simulink model "integratoin_2"  (R2023b)
settings: Solver=FixedStepAuto  StartTime=0.0  StopTime=inf  FixedStep=Ts  RelTol=1e-3
InitFcn:
  | params
  | pin_params
undefined symbols (not defined in the file): b, den_Gd, encoder_scale, f, J, Kb, KD, Kf, KI, Km, KP, l, L, num_Gd, r, R, Vlim, Wref
libraries: arduinolib x29, arduinosensorlib x12, simulink x8
(part 1 of 2)
settings Model: SimulationMode=external  ExtModeTrigDuration=2  Creator=SJ  LastModifiedBy=SJ
settings SolverCC: AutoInsertRateTranBlk=on
settings OptimizationCC: EnhancedBackFolding=on  PassReuseOutputArgsAs=Individual arguments  ZeroExternalMemoryAtStartup=off  ZeroInternalMemoryAtStartup=off  MaxStackSize=64  OptimizeBlockOrder=speed  DifferentSizesBufferReuse=on  OptimizationCustomize=off  EfficientTunableParamExpr=on
settings DebuggingCC: MultiTaskRateTransMsg=warning  ParameterTunabilityLossMsg=error
settings HardwareCC: ProdBitPerInt=16  ProdBitPerPointer=16  ProdBitPerSizeT=16  ProdBitPerPtrDiffT=16  ProdLargestAtomicFloat=None  ProdWordSize=8  ProdHWDeviceType=Atmel->AVR
settings SFSimCC: MATLABDynamicMemAlloc=off
settings RTWCC: Description=Embedded Coder  SystemTargetFile=ert.tlc  HardwareBoard=Arduino Mega 2560  TemplateMakefile=ert_default_tmf  Toolchain=Arduino AVR  BuildConfiguration=Faster Runs
settings CodeAppCC: ForceParamTrailComments=on  IgnoreCustomStorageClasses=off  OperatorAnnotations=on  SimulinkDataObjDesc=on  SFDataObjDesc=on  InsertBlockDesc=on
settings ERTTargetCC: SupportContinuousTime=on  SupportVariableSizeSignals=on  ExtMode=on  ExtModeTransport=3  ExtModeStaticAlloc=on  ExtModeAutomaticAllocSize=off  ExtModeStaticAllocSize=2048  ExtModeMexFile=ext_xcp  ExtModeMexArgs=0 3 921600  ExtModeIntrfLevel=Level2 - Open

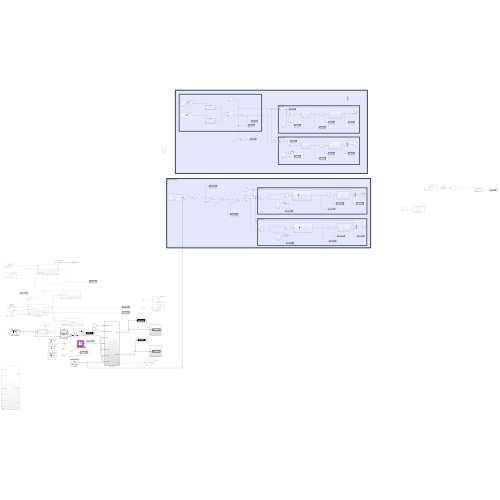
[thumbnail: Simulink's stored preview of the top-level diagram]
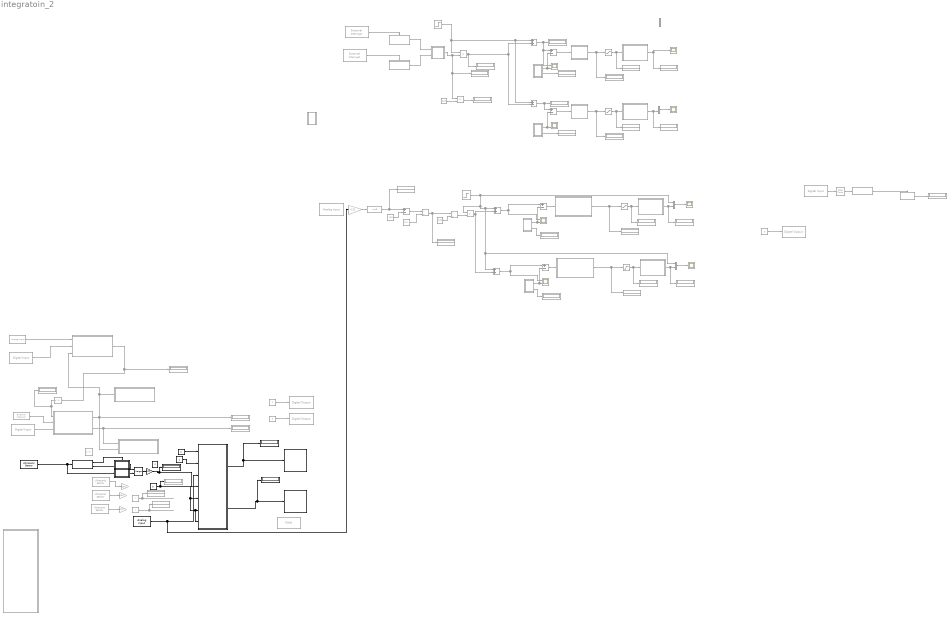
== system integratoin_2 ==
  note: Left Motor
  note: Left Motor
  note: Right Motor
  note: Variable resistance
  note: sw1,2로 1퍼 증가, 감소
  note: Right Motor
  note: 조도 센서 값 * 0.25
      | (평상시 값 800 초반, 손으로 가렸을 때 값 200~300)
  Add : Sum  Commented=on
  Add{1..3,5,7..8} (6 alike) : Sum  Commented=on  Inputs=+-
  Add4 : Sum  Commented=on
  Add6 : Sum  Commented=on
  Analog Input : arduinolib/Analog Input  Commented=on  pinNumber=8  ReadResultsOnly=off  ConversionTriggerSource=Software  ExternalTriggerType=uint32( 0 )  OutputDataType=uint16  EnableConversionCompleteNotify=off  EnableOuputStatus=off  SampleTime=-1  blockPlatform=arduino
  Analog Input1 : arduinolib/Analog Input  Commented=on  pinNumber=BS  ReadResultsOnly=off  ConversionTriggerSource=Software  ExternalTriggerType=uint32( 0 )  OutputDataType=uint16  EnableConversionCompleteNotify=off  EnableOuputStatus=off  SampleTime=-1  blockPlatform=arduino
  Chart : Stateflow chart  Commented=on  TreatAsAtomicUnit=on
  Constant : Constant  Commented=on  Value=128
  Constant1 : Constant  Commented=on  Value=6.4
  Constant10 : Constant  Commented=on  Value=0
  Constant11 : Constant
  Constant12 : Constant
  Constant2 : Constant  Commented=on  Value=100
  Constant3 : Constant  Commented=on  Value=100
  Constant4 : Constant  Value=f
  Constant5 : Constant  Commented=on  Value=0
  Constant6 : Constant  Commented=on  Value=r
  Constant7 : Constant  Value=b
  Constant8 : Constant  Commented=on  Value=l
  Constant9 : Constant  Commented=on
  Data Type Conversion : DataTypeConversion  Commented=on  OutDataTypeStr=uint8  SaturateOnIntegerOverflow=off  RndMeth=Floor
  Delay : Delay  Commented=on  DelayLength=1
  Delay1 : Delay  Commented=on  DelayLength=1
  Digital Input : arduinolib/Digital Input  Commented=on  pinNumber=20  mode=Default  Direction=input  SampleTime=0.1  blockPlatform=arduino
  Digital Input1 : arduinolib/Digital Input  Commented=on  pinNumber=SW3  mode=Default  Direction=input  SampleTime=0.1  blockPlatform=arduino
  Digital Input2 : arduinolib/Digital Input  Commented=on  pinNumber=SW2  mode=Default  Direction=input  SampleTime=0.1  blockPlatform=arduino
  Display{,1..25,29..31,33..34} (31 alike) : Display  Commented=on
  Display27 : Display
  Display28 : Display
  Display32 : Display
  Divide : Product  Commented=on  Inputs=**
  Divide1 : Product  Commented=on  Inputs=*/
  Divide2 : Product  Commented=on  Inputs=**
  Divide3 : Product  Commented=on  Inputs=*/
  Divide4 : Product  Commented=on  Inputs=**
  External Interrupt : arduinolib/External Interrupt  Commented=on  Pin=20  PullUp=off  Mode=FALLING  InterruptSimulationInput=off
  External Interrupt1 : arduinolib/External Interrupt  Commented=on  Pin=21  PullUp=off  Mode=FALLING  InterruptSimulationInput=off
  External Interrupt2 : arduinolib/External Interrupt  Commented=on  Pin=2  PullUp=off  Mode=RISING  InterruptSimulationInput=off
  Function-Call Subsystem1 : Subsystem  Commented=on  TreatAsAtomicUnit=on
  Function-Call Subsystem4 : Subsystem  Commented=on  TreatAsAtomicUnit=on
  Gain : Gain  Commented=on  Gain=0.25
  Gain1 : Gain  Gain=100
  Gain2 : Gain  Commented=on  Gain=100
  Gain3 : Gain  Commented=on  Gain=100
  Gain4 : Gain  Commented=on  Gain=100
  If : If  Commented=on  IfExpression=u1 == 0  ShowElse=off
  If Action Subsystem : Subsystem  Commented=on  TreatAsAtomicUnit=on
  If Action Subsystem1 : Subsystem  TreatAsAtomicUnit=on
  If Action Subsystem2 : Subsystem  TreatAsAtomicUnit=on
  If1 : If  IfExpression=u1 > 1
  LED_B Ctrl : Subsystem  Commented=on
  LED_R Ctrl : Subsystem  Commented=on
  L_Motor(시계) : arduinolib/Digital Output  Commented=on  pinNumber=Motor_L_Direction  Direction=output  blockPlatform=arduino
  Merge : Merge
  Mux{1..4} (4 alike) : Mux  Commented=on  Inputs=2
  PWM1 : arduinolib/PWM  Commented=on  pinNumber=Buzzer  frequencyType=Default  desiredFrequency=490.2  achievableFrequency=490.2
  R_Motor(반시계) : arduinolib/Digital Output  Commented=on  pinNumber=Motor_R_Direction  Direction=output  blockPlatform=arduino
  R_Motor(반시계)1 : arduinolib/Digital Output  Commented=on  pinNumber=Motor_R_Direction  Direction=output  blockPlatform=arduino
  Rate Transition : RateTransition  Commented=on  OutPortSampleTime=0.5
  Saturation{,1..3} (4 alike) : Saturate  Commented=on  UpperLimit=12  LowerLimit=0
  Scope{,1,4,6} (4 alike) : Scope  Commented=on  NumInputPorts=2
  Scope{2..3,5,7} (4 alike) : Scope  Commented=on
  State_Ctrl : Subsystem  Commented=on
  Step : Step  Commented=on  After=Wref  SampleTime=0
  Step1 : Step  Commented=on  After=Wref  SampleTime=0
  Subsystem : Subsystem  Commented=on
  Subsystem1 : Subsystem  Commented=on
  Subsystem10 : Subsystem  Commented=on
  Subsystem11 : Subsystem  Commented=on
  Subsystem12 : Subsystem  Commented=on
  Subsystem13 : Subsystem  Commented=on
  Subsystem14 : Subsystem
  Subsystem15 : Subsystem
  Subsystem16 : Subsystem
  Subsystem2 : Subsystem  Commented=on
  Subsystem3 : Subsystem  Commented=on
  Subsystem4 : Subsystem  Commented=on
  Subsystem5 : Subsystem  Commented=on
  Subsystem6 : Subsystem  Commented=on
  Subsystem7 : Subsystem  Commented=on
  Subsystem8 : Subsystem  Commented=on
  Subsystem9 : Subsystem  Commented=on
  light_Ctrl : Subsystem  Commented=on
  가변저항 : arduinolib/Analog Input  pinNumber=VR  ReadResultsOnly=off  ConversionTriggerSource=Software  ExternalTriggerType=uint32( 0 )  OutputDataType=uint16  EnableConversionCompleteNotify=off  EnableOuputStatus=off  SampleTime=-1  blockPlatform=arduino
  우측 초음파 : arduinosensorlib/Ultrasonic Sensor  Commented=on  NumSignalPins=2  TrigPin=R_Triger  EchoPin=R_Echo  SignalPin=3  SampleTime_=0.1  blockPlatform=ARDUINO
  전방 초음파 : arduinosensorlib/Ultrasonic Sensor  NumSignalPins=2  TrigPin=F_Triger  EchoPin=F_Echo  SignalPin=3  SampleTime_=0.01  blockPlatform=ARDUINO
  좌측 초음파 : arduinosensorlib/Ultrasonic Sensor  Commented=on  NumSignalPins=2  TrigPin=L_Triger  EchoPin=L_Echo  SignalPin=3  SampleTime_=0.1  blockPlatform=ARDUINO
  후방 초음파 : arduinosensorlib/Ultrasonic Sensor  Commented=on  NumSignalPins=2  TrigPin=B_Triger  EchoPin=B_Echo  SignalPin=3  SampleTime_=0.1  blockPlatform=ARDUINO
  wires:
  Subsystem/1(Out1) -> Add1/2, Scope/2
  Saturation/1 -> Subsystem1/1(In2), Display/1
  Subsystem1/1(Out1) -> Scope3/1, Display3/1
  External Interrupt/1 -> Function-Call Subsystem4/Trigger
  External Interrupt1/1 -> Function-Call Subsystem1/Trigger
  Function-Call Subsystem4/1(sw1) -> Chart/1(sw1)
  Function-Call Subsystem1/1(sw2) -> Chart/2(sw2)
  Step/1 -> Divide/1, Add8/1, Add/1
  Divide/1 -> Display1/1, Add/2, Add8/2
  Chart/1(n) -> Divide4/1, Display7/1, Divide/2
  Subsystem/2(Out2) -> Display5/1
  Gain/1 -> Data Type Conversion/1
  Step1/1 -> Mux2/1, Add6/1, Mux3/1, Add4/1, Divide2/1
  Data Type Conversion/1 -> Display12/1, Add2/1
  Constant/1 -> Add2/2
  Divide1/1 -> Display6/1, Divide3/1
  Add2/1 -> Divide1/1
  Constant1/1 -> Divide1/2
  Divide2/1 -> Add6/2, Add4/2
  Constant2/1 -> Divide3/2
  Divide3/1 -> Divide2/2
  Add/1 -> Scope/1, Add1/1, Display4/1
  Saturation1/1 -> Subsystem4/1(In2), Display8/1
  Subsystem3/2(Out2) -> Display11/1
  Subsystem3/1(Out1) -> Add3/2, Scope1/2
  Subsystem4/1(Out1) -> Display10/1, Mux2/2
  Mux2/1 -> Scope2/1
  Add4/1 -> Add3/1, Scope1/1
  Subsystem5/1(Out1) -> Display9/1, Saturation1/1
  Add3/1 -> Subsystem5/1(In1)
  Subsystem6/1(Out1) -> Display2/1, Saturation/1
  Add1/1 -> Subsystem6/1(In1)
  Add6/1 -> Add5/1, Scope4/1
  Mux3/1 -> Scope5/1
  Subsystem7/2(Out2) -> Display14/1
  Subsystem8/1(Out1) -> Display13/1, Mux3/2
  Subsystem7/1(Out1) -> Add5/2, Scope4/2
  Add5/1 -> Subsystem9/1(In1)
  Saturation2/1 -> Subsystem8/1(In2), Display15/1
  Subsystem9/1(Out1) -> Display16/1, Saturation2/1
  Add7/1 -> Subsystem12/1(In1)
  Subsystem11/1(Out1) -> Display19/1, Mux4/2
  Saturation3/1 -> Subsystem11/1(In2), Display17/1
  Mux4/1 -> Scope7/1
  Subsystem10/1(Out1) -> Add7/2, Scope6/2
  Subsystem12/1(Out1) -> Display18/1, Saturation3/1
  Subsystem10/2(Out2) -> Display20/1
  Add8/1 -> Add7/1, Display21/1
  Divide4/1 -> Display22/1
  Constant3/1 -> Divide4/2
  Digital Input/1 -> Rate Transition/1
  If/1 -> If Action Subsystem/Action
  If Action Subsystem/1(Out1) -> Display23/1
  Rate Transition/1 -> If/1
  Constant5/1 -> R_Motor(반시계)/1
  Constant10/1 -> R_Motor(반시계)1/1
  후방 초음파/1 -> Gain2/1
  좌측 초음파/1 -> Gain3/1
  State_Ctrl/1(Drive_mode) -> Display24/1, light_Ctrl/3(Drive_mode1), LED_R Ctrl/1(Drive_mode), LED_B Ctrl/2(Drive_mode)
  Digital Input2/1 -> State_Ctrl/3(SW2)
  Constant9/1 -> L_Motor(시계)/1
  Constant6/1 -> Display29/1
  Analog Input1/1 -> light_Ctrl/1(light1)
  Delay/1 -> Display34/1, State_Ctrl/1(light_mode)
  ? -> PWM1/1
  Digital Input1/1 -> light_Ctrl/2(In2)
  우측 초음파/1 -> Gain4/1
  Constant7/1 -> Subsystem14/7(우측 초음파), Subsystem14/6(좌측 초음파), Subsystem14/5(전방 초음파), Display31/1
  State_Ctrl/2(ADAS_state1) -> LED_B Ctrl/1(ADAS_state), Display25/1
  Constant8/1 -> Display30/1
  가변저항/1 -> Subsystem14/3(가변저항), Gain/1
  External Interrupt2/1 -> State_Ctrl/2(SW1)
  light_Ctrl/1(light_mode) -> Display33/1, Delay/1
  Constant11/1 -> Subsystem14/1(DRIVE MODE)
  Constant12/1 -> Subsystem14/2(ADAS MODE)
  If1/1 -> If Action Subsystem1/Action
  If Action Subsystem1/1(Out1) -> Merge/1
  Merge/1 -> Gain1/1
  If1/2 -> If Action Subsystem2/Action
  If Action Subsystem2/1(Out1) -> Merge/2
  Subsystem14/1(L_Motor) -> Subsystem15/1(L_Motor), Display27/1
  Subsystem14/2(R_Motor) -> Display28/1, Subsystem16/1(L_Motor)
  Gain1/1 -> Subsystem14/4(In1), Display32/1
  ? -> ?
  ? -> ?
  전방 초음파/1 -> If Action Subsystem2/1(In1), If1/1

== system integratoin_2/Function-Call Subsystem1 ==
  function : TriggerPort  TriggerType=function-call  VariantControl=(inherit)
  Add : Sum  Inputs=+-
  Constant : Constant
  Delay : Delay  DelayLength=1
  sw2 : Outport
  wires:
  Add/1 -> Delay/1, sw2/1
  Delay/1 -> Add/2
  Constant/1 -> Add/1

== system integratoin_2/Function-Call Subsystem4 ==
  function : TriggerPort  TriggerType=function-call  VariantControl=(inherit)
  Add : Sum  Inputs=+-
  Constant : Constant
  Delay : Delay  DelayLength=1
  sw1 : Outport
  wires:
  Add/1 -> sw1/1, Delay/1
  Delay/1 -> Add/2
  Constant/1 -> Add/1

== system integratoin_2/If Action Subsystem ==
  Action Port : ActionPort  ActionPortLabel=if(u1 == 0)
  Add : Sum
  Constant : Constant
  Constant1 : Constant  Value=3
  Delay : Delay  DelayLength=1
  Mod : Math  Operator=mod
  Out1 : Outport
  wires:
  Mod/1 -> Delay/1, Out1/1
  Delay/1 -> Add/2
  Constant/1 -> Add/1
  Add/1 -> Mod/1
  Constant1/1 -> Mod/2

== system integratoin_2/If Action Subsystem1 ==
  Action Port : ActionPort  ActionPortLabel=if(u1 > 1)
  Constant : Constant
  Out1 : Outport
  wires:
  Constant/1 -> Out1/1

== system integratoin_2/If Action Subsystem2 ==
  In1 : Inport
  Action Port : ActionPort  ActionPortLabel=else
  Out1 : Outport
  wires:
  In1/1 -> Out1/1

== system integratoin_2/LED_B Ctrl ==
  ADAS_state : Inport
  Drive_mode : Inport  Port=2
  Constant : Constant
  Digital Output : arduinolib/Digital Output  pinNumber=LED1_B  Direction=output  blockPlatform=arduino
  If Action Subsystem1 : Subsystem  TreatAsAtomicUnit=on
  If Action Subsystem3 : Subsystem  TreatAsAtomicUnit=on
  If1 : If  IfExpression=u1 ==1
  Merge : Merge
  Product : Product
  Product1 : Product
  Pulse Generator : DiscretePulseGenerator  PulseType=Time based  PulseWidth=50
  wires:
  If1/2 -> If Action Subsystem3/Action
  If Action Subsystem1/1(Out1) -> Merge/1
  ADAS_state/1 -> If1/1
  If1/1 -> If Action Subsystem1/Action
  Merge/1 -> Digital Output/1
  If Action Subsystem3/1(Out1) -> Merge/2
  Drive_mode/1 -> Product/1, Product1/2
  Pulse Generator/1 -> Product/2
  Constant/1 -> Product1/1
  Product1/1 -> If Action Subsystem1/1(Input)
  Product/1 -> If Action Subsystem3/1(Input)

== system integratoin_2/LED_R Ctrl ==
  Drive_mode : Inport
  Digital Output : arduinolib/Digital Output  pinNumber=LED1_R  Direction=output  blockPlatform=arduino
  If Action Subsystem1 : Subsystem  TreatAsAtomicUnit=on
  If Action Subsystem3 : Subsystem  TreatAsAtomicUnit=on
  If1 : If  IfExpression=u1 ==1
  Merge : Merge
  wires:
  If1/2 -> If Action Subsystem3/Action
  If Action Subsystem1/1(Out1) -> Merge/1
  Drive_mode/1 -> If1/1
  If1/1 -> If Action Subsystem1/Action
  Merge/1 -> Digital Output/1
  If Action Subsystem3/1(Out1) -> Merge/2

== system integratoin_2/State_Ctrl ==
  light_mode : Inport
  SW1 : Inport  Port=2
  SW2 : Inport  Port=3
  ADAS_state : Subsystem
  Delay : Delay  DelayLength=1
  If : If  IfExpression=u1 ==1  ShowElse=off
  Rate Transition2 : RateTransition  Integrity=off  OutPortSampleTime=0.2
  drive_mode : Subsystem
  Drive_mode : Outport
  ADAS_state1 : Outport  Port=2
  wires:
  If/1 -> ADAS_state/1(In1)
  drive_mode/1(D_mode) -> If/1, Drive_mode/1
  ADAS_state/1(ADAS_state) -> Delay/1, ADAS_state1/1
  SW1/1 -> drive_mode/2(sw1)
  Delay/1 -> drive_mode/3(A_state)
  light_mode/1 -> drive_mode/1(light_mode)
  SW2/1 -> Rate Transition2/1
  Rate Transition2/1 -> ADAS_state/2(In2)

== system integratoin_2/Subsystem ==
  Data Type Conversion1 : DataTypeConversion  OutDataTypeStr=int32  SaturateOnIntegerOverflow=off  RndMeth=Floor
  Discrete Transfer Fcn : DiscreteTransferFcn  Numerator=num_Gd  Denominator=den_Gd
  Discrete Derivative : simulink/Discrete/Discrete Derivative  gainval=1.0  ICPrevScaledInput=0.0  OutMin=[]  OutMax=[]  OutDataType=fixdt(1, 16)  OutScaling=2^-10  DoSatur=off
  Display : Display
  Encoder : arduinosensorlib/Encoder  InputA=18  InputB=19  Mode=No reset  SampleTime=-1
  Gain1 : Gain  Gain=encoder_scale
  Gain2 : Gain  Gain=60/(2*pi)
  Out1 : Outport
  Out2 : Outport  Port=2
  wires:
  Gain1/1 -> Display/1, Gain2/1, Data Type Conversion1/1
  Encoder/1 -> Discrete Derivative/1
  Gain2/1 -> Out2/1
  Data Type Conversion1/1 -> Discrete Transfer Fcn/1
  Discrete Derivative/1 -> Gain1/1
  Discrete Transfer Fcn/1 -> Out1/1

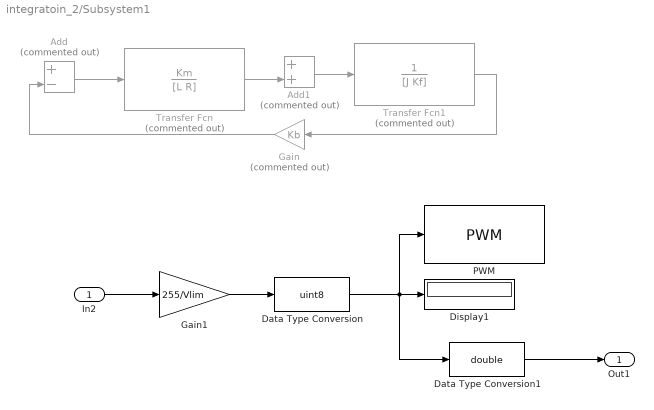
== system integratoin_2/Subsystem1 ==
  In2 : Inport
  Add : Sum  Commented=on  Inputs=+-
  Add1 : Sum  Commented=on
  Data Type Conversion : DataTypeConversion  OutDataTypeStr=uint8  SaturateOnIntegerOverflow=off  RndMeth=Floor
  Data Type Conversion1 : DataTypeConversion  OutDataTypeStr=double  SaturateOnIntegerOverflow=off  RndMeth=Floor
  Display1 : Display
  Gain : Gain  Commented=on  Gain=Kb
  Gain1 : Gain  Gain=255/Vlim
  PWM : arduinolib/PWM  pinNumber=11  frequencyType=Default  desiredFrequency=490.2  achievableFrequency=490.2
  Transfer Fcn : TransferFcn  Commented=on  Numerator=Km  Denominator=[L R]
  Transfer Fcn1 : TransferFcn  Commented=on  Numerator=1  Denominator=[J Kf]
  Out1 : Outport
  wires:
  ? -> Add/1
  ? -> Add1/1
  Add/1 -> Transfer Fcn/1
  Add1/1 -> Transfer Fcn1/1
  Transfer Fcn/1 -> Add1/2
  Gain/1 -> Add/2
  Transfer Fcn1/1 -> Gain/1
  In2/1 -> Gain1/1
  Gain1/1 -> Data Type Conversion/1
  Data Type Conversion1/1 -> Out1/1
  Data Type Conversion/1 -> Data Type Conversion1/1, Display1/1, PWM/1

== system integratoin_2/Subsystem10 ==
  Data Type Conversion1 : DataTypeConversion  OutDataTypeStr=int32  SaturateOnIntegerOverflow=off  RndMeth=Floor
  Discrete Transfer Fcn : DiscreteTransferFcn  Numerator=num_Gd  Denominator=den_Gd
  Discrete Derivative : simulink/Discrete/Discrete Derivative  gainval=1.0  ICPrevScaledInput=0.0  OutMin=[]  OutMax=[]  OutDataType=fixdt(1, 16)  OutScaling=2^-10  DoSatur=off
  Display : Display
  Encoder : arduinosensorlib/Encoder  InputA=20  InputB=21  Mode=No reset  SampleTime=-1
  Gain1 : Gain  Gain=encoder_scale
  Gain2 : Gain  Gain=60/(2*pi)
  Out1 : Outport
  Out2 : Outport  Port=2
  wires:
  Gain1/1 -> Display/1, Gain2/1, Data Type Conversion1/1
  Encoder/1 -> Discrete Derivative/1
  Gain2/1 -> Out2/1
  Data Type Conversion1/1 -> Discrete Transfer Fcn/1
  Discrete Derivative/1 -> Gain1/1
  Discrete Transfer Fcn/1 -> Out1/1

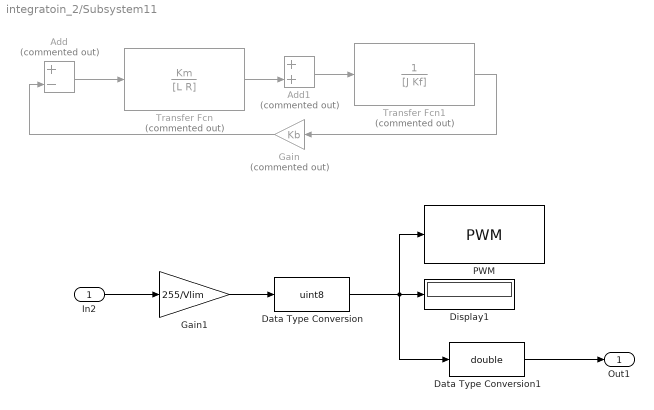
== system integratoin_2/Subsystem11 ==
  In2 : Inport
  Add : Sum  Commented=on  Inputs=+-
  Add1 : Sum  Commented=on
  Data Type Conversion : DataTypeConversion  OutDataTypeStr=uint8  SaturateOnIntegerOverflow=off  RndMeth=Floor
  Data Type Conversion1 : DataTypeConversion  OutDataTypeStr=double  SaturateOnIntegerOverflow=off  RndMeth=Floor
  Display1 : Display
  Gain : Gain  Commented=on  Gain=Kb
  Gain1 : Gain  Gain=255/Vlim
  PWM : arduinolib/PWM  pinNumber=11  frequencyType=Default  desiredFrequency=490.2  achievableFrequency=490.2
  Transfer Fcn : TransferFcn  Commented=on  Numerator=Km  Denominator=[L R]
  Transfer Fcn1 : TransferFcn  Commented=on  Numerator=1  Denominator=[J Kf]
  Out1 : Outport
  wires:
  ? -> Add/1
  ? -> Add1/1
  Add/1 -> Transfer Fcn/1
  Add1/1 -> Transfer Fcn1/1
  Transfer Fcn/1 -> Add1/2
  Gain/1 -> Add/2
  Transfer Fcn1/1 -> Gain/1
  In2/1 -> Gain1/1
  Gain1/1 -> Data Type Conversion/1
  Data Type Conversion1/1 -> Out1/1
  Data Type Conversion/1 -> Data Type Conversion1/1, Display1/1, PWM/1

== system integratoin_2/Subsystem12 ==
  In1 : Inport
  Derivative1 : Derivative  Commented=on
  Gain4 : Gain  Commented=on  Gain=KI
  Gain5 : Gain  Commented=on  Gain=KP
  Gain6 : Gain  Commented=on  Gain=KD
  Integrator1 : Integrator  Commented=on
  Subtract1 : Sum  Commented=on  Inputs=+++
  Out1 : Outport
  wires:
  Derivative1/1 -> Subtract1/3
  Gain4/1 -> Integrator1/1
  Integrator1/1 -> Subtract1/1
  Gain6/1 -> Derivative1/1
  Subtract1/1 -> Out1/1
  In1/1 -> Gain5/1, Gain6/1, Gain4/1
  Gain5/1 -> Subtract1/2

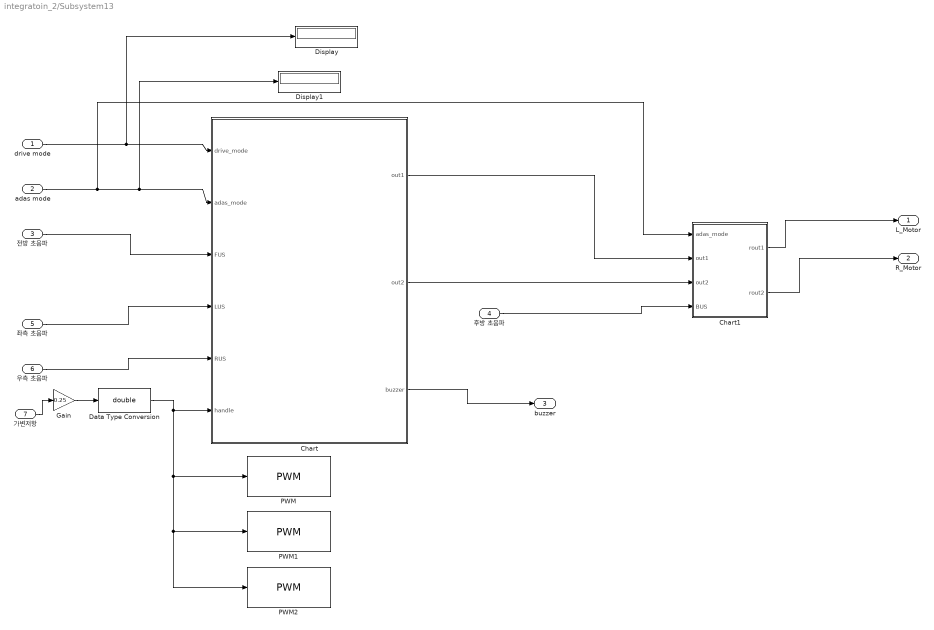
== system integratoin_2/Subsystem13 ==
  drive mode : Inport
  adas mode : Inport  Port=2
  전방 초음파 : Inport  Port=3
  후방 초음파 : Inport  Port=4
  좌측 초음파 : Inport  Port=5
  우측 초음파 : Inport  Port=6
  가변저항 : Inport  Port=7
  Chart : Stateflow chart  TreatAsAtomicUnit=on
  Chart1 : Stateflow chart  TreatAsAtomicUnit=on
  Data Type Conversion : DataTypeConversion  OutDataTypeStr=double  SaturateOnIntegerOverflow=off  RndMeth=Floor
  Display : Display
  Display1 : Display
  Gain : Gain  Gain=0.25
  PWM : arduinolib/PWM  pinNumber=RGB_LED_1  frequencyType=Default  desiredFrequency=490.2  achievableFrequency=490.2
  PWM1 : arduinolib/PWM  pinNumber=RGB_LED_2  frequencyType=Default  desiredFrequency=490.2  achievableFrequency=490.2
  PWM2 : arduinolib/PWM  pinNumber=RGB_LED_3  frequencyType=Default  desiredFrequency=490.2  achievableFrequency=490.2
  L_Motor : Outport
  R_Motor : Outport  Port=2
  buzzer : Outport  Port=3
  wires:
  drive mode/1 -> Chart/1(drive_mode), Display/1
  adas mode/1 -> Chart1/1(adas_mode), Chart/2(adas_mode), Display1/1
  전방 초음파/1 -> Chart/3(FUS)
  후방 초음파/1 -> Chart1/4(BUS)
  좌측 초음파/1 -> Chart/4(LUS)
  우측 초음파/1 -> Chart/5(RUS)
  Chart/3(buzzer) -> buzzer/1
  Chart/1(out1) -> Chart1/2(out1)
  Chart/2(out2) -> Chart1/3(out2)
  Chart1/1(rout1) -> L_Motor/1
  Chart1/2(rout2) -> R_Motor/1
  가변저항/1 -> Gain/1
  Gain/1 -> Data Type Conversion/1
  Data Type Conversion/1 -> PWM2/1, PWM1/1, PWM/1, Chart/6(handle)

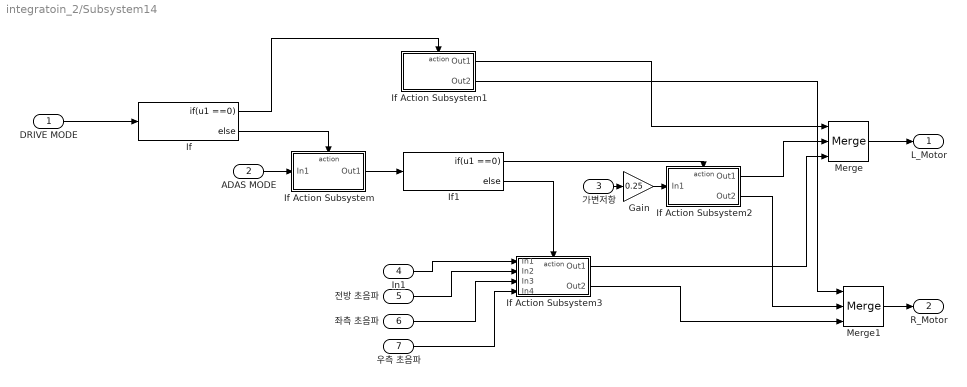
== system integratoin_2/Subsystem14 ==
  DRIVE MODE : Inport
  ADAS MODE : Inport  Port=2
  가변저항 : Inport  Port=3
  In1 : Inport  Port=4
  전방 초음파 : Inport  Port=5
  좌측 초음파 : Inport  Port=6
  우측 초음파 : Inport  Port=7
  Gain : Gain  Gain=0.25
  If : If  IfExpression=u1 ==0
  If Action Subsystem : Subsystem  TreatAsAtomicUnit=on
  If Action Subsystem1 : Subsystem  TreatAsAtomicUnit=on
  If Action Subsystem2 : Subsystem  TreatAsAtomicUnit=on
  If Action Subsystem3 : Subsystem  TreatAsAtomicUnit=on
  If1 : If  IfExpression=u1 ==0
  Merge : Merge  Inputs=3
  Merge1 : Merge  Inputs=3
  L_Motor : Outport
  R_Motor : Outport  Port=2
  wires:
  DRIVE MODE/1 -> If/1
  If/2 -> If Action Subsystem/Action
  If/1 -> If Action Subsystem1/Action
  ADAS MODE/1 -> If Action Subsystem/1(In1)
  If Action Subsystem/1(Out1) -> If1/1
  If1/1 -> If Action Subsystem2/Action
  If1/2 -> If Action Subsystem3/Action
  In1/1 -> If Action Subsystem3/1(In1)
  전방 초음파/1 -> If Action Subsystem3/2(In2)
  좌측 초음파/1 -> If Action Subsystem3/3(In3)
  우측 초음파/1 -> If Action Subsystem3/4(In4)
  If Action Subsystem1/1(Out1) -> Merge/1
  If Action Subsystem2/1(Out1) -> Merge/2
  If Action Subsystem3/1(Out1) -> Merge/3
  If Action Subsystem1/2(Out2) -> Merge1/1
  If Action Subsystem2/2(Out2) -> Merge1/2
  If Action Subsystem3/2(Out2) -> Merge1/3
  Merge/1 -> L_Motor/1
  Merge1/1 -> R_Motor/1
  가변저항/1 -> Gain/1
  Gain/1 -> If Action Subsystem2/1(In1)

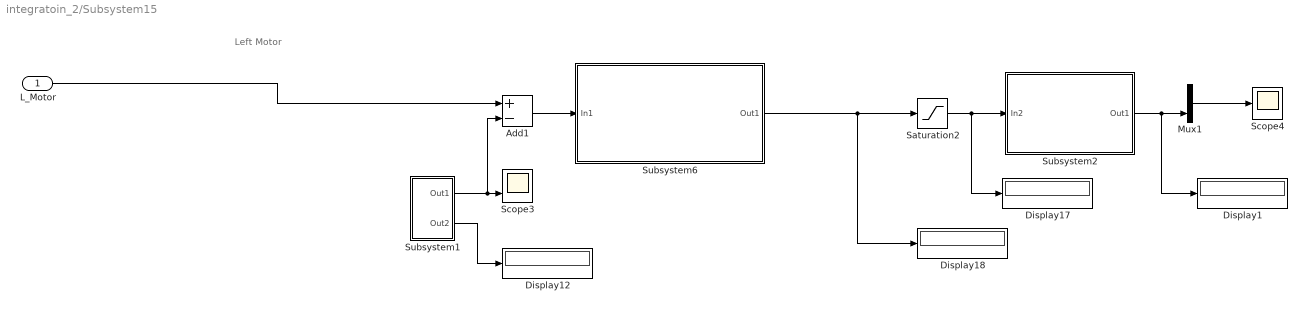
== system integratoin_2/Subsystem15 ==
  note: Left Motor
  L_Motor : Inport
  Add1 : Sum  Inputs=+-
  Display{1,12,17..18} (4 alike) : Display
  Mux1 : Mux  Inputs=2
  Saturation2 : Saturate  UpperLimit=12  LowerLimit=0
  Scope3 : Scope  NumInputPorts=2
  Scope4 : Scope
  Subsystem1 : Subsystem
  Subsystem2 : Subsystem
  Subsystem6 : Subsystem
  wires:
  Subsystem2/1(Out1) -> Display1/1, Mux1/2
  Subsystem1/2(Out2) -> Display12/1
  Subsystem6/1(Out1) -> Display18/1, Saturation2/1
  Add1/1 -> Subsystem6/1(In1)
  Mux1/1 -> Scope4/1
  Subsystem1/1(Out1) -> Add1/2, Scope3/2
  Saturation2/1 -> Subsystem2/1(In2), Display17/1
  L_Motor/1 -> Add1/1

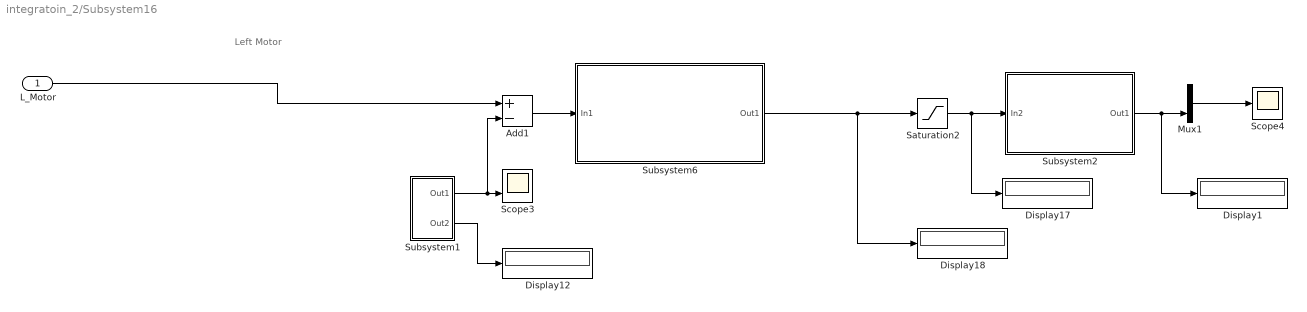
== system integratoin_2/Subsystem16 ==
  note: Left Motor
  L_Motor : Inport
  Add1 : Sum  Inputs=+-
  Display{1,12,17..18} (4 alike) : Display
  Mux1 : Mux  Inputs=2
  Saturation2 : Saturate  UpperLimit=12  LowerLimit=0
  Scope3 : Scope  NumInputPorts=2
  Scope4 : Scope
  Subsystem1 : Subsystem
  Subsystem2 : Subsystem
  Subsystem6 : Subsystem
  wires:
  Subsystem2/1(Out1) -> Display1/1, Mux1/2
  Subsystem1/2(Out2) -> Display12/1
  Subsystem6/1(Out1) -> Display18/1, Saturation2/1
  Add1/1 -> Subsystem6/1(In1)
  Mux1/1 -> Scope4/1
  Subsystem1/1(Out1) -> Add1/2, Scope3/2
  Saturation2/1 -> Subsystem2/1(In2), Display17/1
  L_Motor/1 -> Add1/1
  ? -> Scope3/1

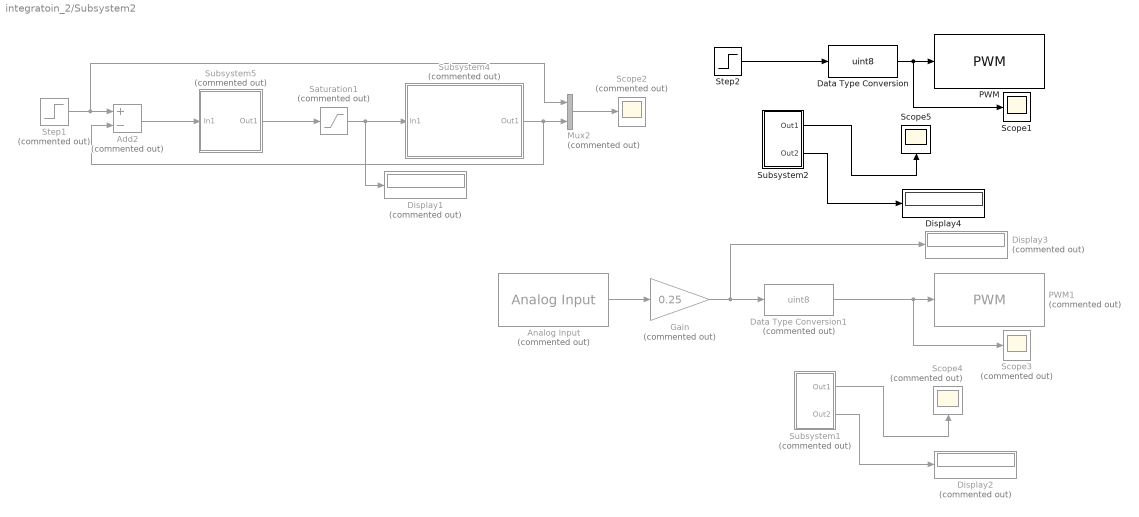
== system integratoin_2/Subsystem2 ==
  Add2 : Sum  Commented=on  Inputs=+-
  Analog Input : arduinolib/Analog Input  Commented=on  pinNumber=8  ReadResultsOnly=off  ConversionTriggerSource=Software  ExternalTriggerType=uint32( 0 )  OutputDataType=uint16  EnableConversionCompleteNotify=off  EnableOuputStatus=off  SampleTime=-1  blockPlatform=arduino
  Data Type Conversion : DataTypeConversion  OutDataTypeStr=uint8  SaturateOnIntegerOverflow=off  RndMeth=Floor
  Data Type Conversion1 : DataTypeConversion  Commented=on  OutDataTypeStr=uint8  SaturateOnIntegerOverflow=off  RndMeth=Floor
  Display1 : Display  Commented=on
  Display2 : Display  Commented=on
  Display3 : Display  Commented=on
  Display4 : Display
  Gain : Gain  Commented=on  Gain=0.25
  Mux2 : Mux  Commented=on  Inputs=2
  PWM : arduinolib/PWM  pinNumber=11  frequencyType=Default  desiredFrequency=490.2  achievableFrequency=490.2
  PWM1 : arduinolib/PWM  Commented=on  pinNumber=11  frequencyType=Default  desiredFrequency=490.2  achievableFrequency=490.2
  Saturation1 : Saturate  Commented=on  UpperLimit=Vlim  LowerLimit=0
  Scope1 : Scope
  Scope2 : Scope  Commented=on
  Scope3 : Scope  Commented=on
  Scope4 : Scope  Commented=on
  Scope5 : Scope
  Step1 : Step  Commented=on  After=Wref  SampleTime=0
  Step2 : Step  After=Wref  SampleTime=0
  Subsystem1 : Subsystem  Commented=on
  Subsystem2 : Subsystem
  Subsystem4 : Subsystem  Commented=on
  Subsystem5 : Subsystem  Commented=on
  wires:
  Data Type Conversion/1 -> Scope1/1, PWM/1
  Add2/1 -> Subsystem5/1(In1)
  Saturation1/1 -> Subsystem4/1(In1), Display1/1
  Mux2/1 -> Scope2/1
  Subsystem4/1(Out1) -> Add2/2, Mux2/2
  Step2/1 -> Data Type Conversion/1
  Subsystem5/1(Out1) -> Saturation1/1
  Step1/1 -> Mux2/1, Add2/1
  Subsystem1/1(Out1) -> Scope4/1
  Gain/1 -> Display3/1, Data Type Conversion1/1
  Data Type Conversion1/1 -> Scope3/1, PWM1/1
  Analog Input/1 -> Gain/1
  Subsystem1/2(Out2) -> Display2/1
  Subsystem2/1(Out1) -> Scope5/1
  Subsystem2/2(Out2) -> Display4/1

== system integratoin_2/Subsystem3 ==
  Data Type Conversion1 : DataTypeConversion  OutDataTypeStr=int32  SaturateOnIntegerOverflow=off  RndMeth=Floor
  Discrete Transfer Fcn : DiscreteTransferFcn  Numerator=num_Gd  Denominator=den_Gd
  Discrete Derivative : simulink/Discrete/Discrete Derivative  gainval=1.0  ICPrevScaledInput=0.0  OutMin=[]  OutMax=[]  OutDataType=fixdt(1, 16)  OutScaling=2^-10  DoSatur=off
  Display : Display
  Encoder : arduinosensorlib/Encoder  InputA=18  InputB=19  Mode=No reset  SampleTime=-1
  Gain1 : Gain  Gain=encoder_scale
  Gain2 : Gain  Gain=60/(2*pi)
  Out1 : Outport
  Out2 : Outport  Port=2
  wires:
  Gain1/1 -> Display/1, Gain2/1, Data Type Conversion1/1
  Encoder/1 -> Discrete Derivative/1
  Gain2/1 -> Out2/1
  Data Type Conversion1/1 -> Discrete Transfer Fcn/1
  Discrete Derivative/1 -> Gain1/1
  Discrete Transfer Fcn/1 -> Out1/1

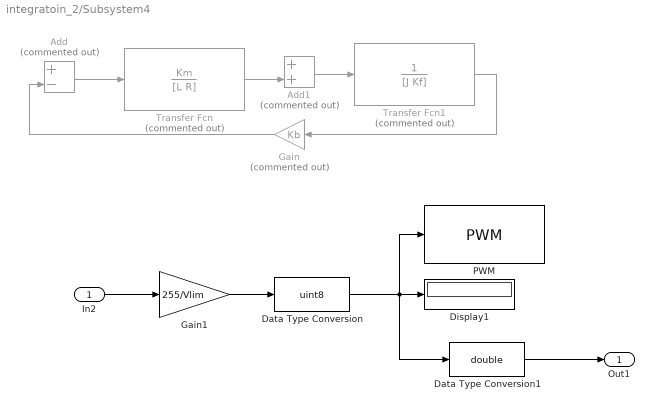
== system integratoin_2/Subsystem4 ==
  In2 : Inport
  Add : Sum  Commented=on  Inputs=+-
  Add1 : Sum  Commented=on
  Data Type Conversion : DataTypeConversion  OutDataTypeStr=uint8  SaturateOnIntegerOverflow=off  RndMeth=Floor
  Data Type Conversion1 : DataTypeConversion  OutDataTypeStr=double  SaturateOnIntegerOverflow=off  RndMeth=Floor
  Display1 : Display
  Gain : Gain  Commented=on  Gain=Kb
  Gain1 : Gain  Gain=255/Vlim
  PWM : arduinolib/PWM  pinNumber=11  frequencyType=Default  desiredFrequency=490.2  achievableFrequency=490.2
  Transfer Fcn : TransferFcn  Commented=on  Numerator=Km  Denominator=[L R]
  Transfer Fcn1 : TransferFcn  Commented=on  Numerator=1  Denominator=[J Kf]
  Out1 : Outport
  wires:
  ? -> Add/1
  ? -> Add1/1
  Add/1 -> Transfer Fcn/1
  Add1/1 -> Transfer Fcn1/1
  Transfer Fcn/1 -> Add1/2
  Gain/1 -> Add/2
  Transfer Fcn1/1 -> Gain/1
  In2/1 -> Gain1/1
  Gain1/1 -> Data Type Conversion/1
  Data Type Conversion1/1 -> Out1/1
  Data Type Conversion/1 -> Data Type Conversion1/1, Display1/1, PWM/1

== system integratoin_2/Subsystem5 ==
  In1 : Inport
  Derivative2 : Derivative
  Gain1 : Gain  Gain=KI
  Gain2 : Gain  Gain=KP
  Gain3 : Gain  Gain=KD
  Integrator2 : Integrator
  Subtract2 : Sum  Inputs=+++
  Out1 : Outport
  wires:
  Gain1/1 -> Integrator2/1
  Gain2/1 -> Subtract2/2
  Integrator2/1 -> Subtract2/1
  In1/1 -> Gain2/1, Gain3/1, Gain1/1
  Derivative2/1 -> Subtract2/3
  Gain3/1 -> Derivative2/1
  Subtract2/1 -> Out1/1

== system integratoin_2/Subsystem6 ==
  In1 : Inport
  Derivative1 : Derivative
  Gain4 : Gain  Gain=KI
  Gain5 : Gain  Gain=KP
  Gain6 : Gain  Gain=KD
  Integrator1 : Integrator
  Subtract1 : Sum  Inputs=+++
  Out1 : Outport
  wires:
  Derivative1/1 -> Subtract1/3
  Gain4/1 -> Integrator1/1
  Integrator1/1 -> Subtract1/1
  Gain6/1 -> Derivative1/1
  Subtract1/1 -> Out1/1
  In1/1 -> Gain5/1, Gain6/1, Gain4/1
  Gain5/1 -> Subtract1/2

== system integratoin_2/Subsystem7 ==
  Data Type Conversion1 : DataTypeConversion  OutDataTypeStr=int32  SaturateOnIntegerOverflow=off  RndMeth=Floor
  Discrete Transfer Fcn : DiscreteTransferFcn  Numerator=num_Gd  Denominator=den_Gd
  Discrete Derivative : simulink/Discrete/Discrete Derivative  gainval=1.0  ICPrevScaledInput=0.0  OutMin=[]  OutMax=[]  OutDataType=fixdt(1, 16)  OutScaling=2^-10  DoSatur=off
  Display : Display
  Encoder : arduinosensorlib/Encoder  InputA=20  InputB=21  Mode=No reset  SampleTime=-1
  Gain1 : Gain  Gain=encoder_scale
  Gain2 : Gain  Gain=60/(2*pi)
  Out1 : Outport
  Out2 : Outport  Port=2
  wires:
  Gain1/1 -> Display/1, Gain2/1, Data Type Conversion1/1
  Encoder/1 -> Discrete Derivative/1
  Gain2/1 -> Out2/1
  Data Type Conversion1/1 -> Discrete Transfer Fcn/1
  Discrete Derivative/1 -> Gain1/1
  Discrete Transfer Fcn/1 -> Out1/1

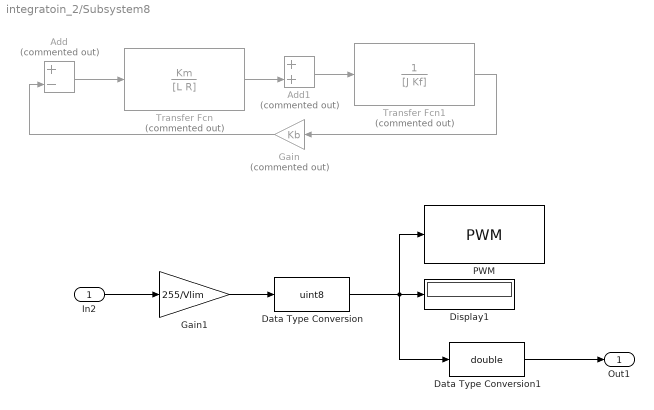
== system integratoin_2/Subsystem8 ==
  In2 : Inport
  Add : Sum  Commented=on  Inputs=+-
  Add1 : Sum  Commented=on
  Data Type Conversion : DataTypeConversion  OutDataTypeStr=uint8  SaturateOnIntegerOverflow=off  RndMeth=Floor
  Data Type Conversion1 : DataTypeConversion  OutDataTypeStr=double  SaturateOnIntegerOverflow=off  RndMeth=Floor
  Display1 : Display
  Gain : Gain  Commented=on  Gain=Kb
  Gain1 : Gain  Gain=255/Vlim
  PWM : arduinolib/PWM  pinNumber=3  frequencyType=Default  desiredFrequency=490.2  achievableFrequency=490.2
  Transfer Fcn : TransferFcn  Commented=on  Numerator=Km  Denominator=[L R]
  Transfer Fcn1 : TransferFcn  Commented=on  Numerator=1  Denominator=[J Kf]
  Out1 : Outport
  wires:
  ? -> Add/1
  ? -> Add1/1
  Add/1 -> Transfer Fcn/1
  Add1/1 -> Transfer Fcn1/1
  Transfer Fcn/1 -> Add1/2
  Gain/1 -> Add/2
  Transfer Fcn1/1 -> Gain/1
  In2/1 -> Gain1/1
  Gain1/1 -> Data Type Conversion/1
  Data Type Conversion1/1 -> Out1/1
  Data Type Conversion/1 -> Data Type Conversion1/1, Display1/1, PWM/1

== system integratoin_2/Subsystem9 ==
  In1 : Inport
  Derivative2 : Derivative
  Gain1 : Gain  Gain=KI
  Gain2 : Gain  Gain=KP
  Gain3 : Gain  Gain=KD
  Integrator2 : Integrator
  Subtract2 : Sum  Inputs=+++
  Out1 : Outport
  wires:
  Gain1/1 -> Integrator2/1
  Gain2/1 -> Subtract2/2
  Integrator2/1 -> Subtract2/1
  In1/1 -> Gain2/1, Gain3/1, Gain1/1
  Derivative2/1 -> Subtract2/3
  Gain3/1 -> Derivative2/1
  Subtract2/1 -> Out1/1

== system integratoin_2/light_Ctrl ==
  light1 : Inport
  In2 : Inport  Port=2
  Drive_mode1 : Inport  Port=3
  Display1 : Display
  Function-Call Subsystem1 : Subsystem  Commented=on  TreatAsAtomicUnit=on
  If : If  IfExpression=u1 == 0  ShowElse=off
  If Action Subsystem : Subsystem  TreatAsAtomicUnit=on
  Rate Transition : RateTransition  Integrity=off
  Rate Transition1 : RateTransition  Integrity=off  OutPortSampleTime=0.2
  Subsystem : Subsystem
  light_mode : Outport
  wires:
  If Action Subsystem/1(Out1) -> Display1/1, Rate Transition/1
  In2/1 -> Rate Transition1/1
  Rate Transition/1 -> Subsystem/2(sw3)
  Drive_mode1/1 -> Subsystem/3(Drive_mode1)
  light1/1 -> Subsystem/1(light1)
  Subsystem/1(light_mode) -> light_mode/1
  If/1 -> If Action Subsystem/Action
  Rate Transition1/1 -> If/1

== system integratoin_2/LED_B Ctrl/If Action Subsystem1 ==
  Input : Inport
  Action Port : ActionPort  ActionPortLabel=if(u1 ==1)
  Out1 : Outport
  wires:
  Input/1 -> Out1/1

== system integratoin_2/LED_B Ctrl/If Action Subsystem3 ==
  Input : Inport
  Action Port : ActionPort  ActionPortLabel=else
  Out1 : Outport
  wires:
  Input/1 -> Out1/1

== system integratoin_2/LED_R Ctrl/If Action Subsystem1 ==
  Action Port : ActionPort  ActionPortLabel=if(u1 ==1)
  Constant : Constant
  Out1 : Outport
  wires:
  Constant/1 -> Out1/1

== system integratoin_2/LED_R Ctrl/If Action Subsystem3 ==
  Action Port : ActionPort  ActionPortLabel=else
  Constant : Constant  Value=0
  Out1 : Outport
  wires:
  Constant/1 -> Out1/1

== system integratoin_2/State_Ctrl/ADAS_state ==
  In1 : Inport
  In2 : Inport  Port=2
  If : If  IfExpression=u1 == 0  ShowElse=off
  If Action Subsystem : Subsystem  TreatAsAtomicUnit=on
  If Action Subsystem1 : Subsystem  TreatAsAtomicUnit=on
  Rate Transition2 : RateTransition  Integrity=off  OutPortSampleTime=0.2
  SW2 : Subsystem  Commented=on
  ADAS_state : Outport
  wires:
  In1/1 -> If Action Subsystem/Action
  If Action Subsystem/1(ADAS_state) -> ADAS_state/1
  In2/1 -> Rate Transition2/1
  Rate Transition2/1 -> If/1
  If/1 -> If Action Subsystem1/Action
  If Action Subsystem1/1(sw2) -> If Action Subsystem/1(sw2)

== system integratoin_2/State_Ctrl/drive_mode ==
  light_mode : Inport
  sw1 : Inport  Port=2
  A_state : Inport  Port=3
  Chart : Stateflow chart  TreatAsAtomicUnit=on
  Rate Transition : RateTransition  Integrity=off
  SW1 : Subsystem
  D_mode : Outport
  wires:
  SW1/1(Output) -> Rate Transition/1
  Rate Transition/1 -> Chart/1(sw1)
  Chart/1(drive_mode) -> D_mode/1
  sw1/1 -> SW1/Trigger
  A_state/1 -> Chart/3(A_state)
  light_mode/1 -> Chart/2(light_mode)

== system integratoin_2/Subsystem14/If Action Subsystem ==
  In1 : Inport
  Action Port : ActionPort  ActionPortLabel=else
  Out1 : Outport
  wires:
  In1/1 -> Out1/1

== system integratoin_2/Subsystem14/If Action Subsystem1 ==
  Action Port : ActionPort  ActionPortLabel=if(u1 ==0)
  Constant : Constant  Value=0
  Constant1 : Constant  Value=0
  Out1 : Outport
  Out2 : Outport  Port=2
  wires:
  Constant/1 -> Out1/1
  Constant1/1 -> Out2/1

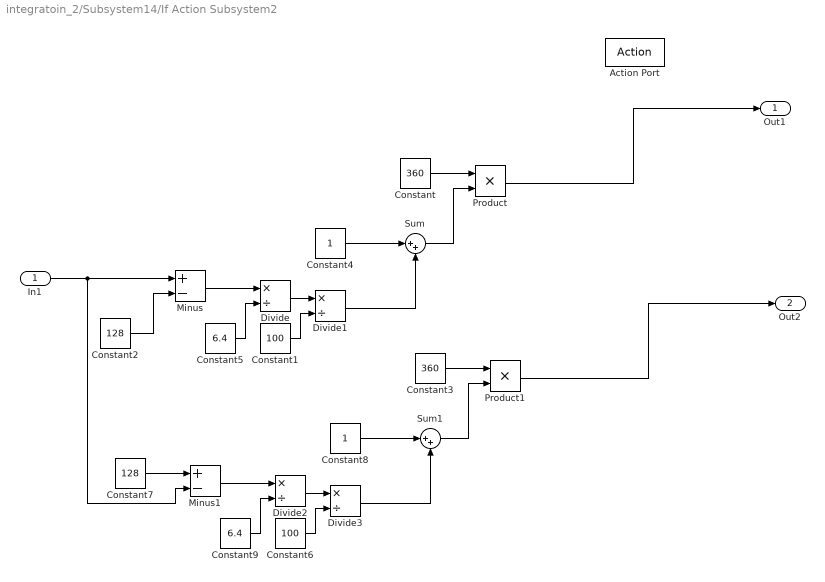
== system integratoin_2/Subsystem14/If Action Subsystem2 ==
  In1 : Inport
  Action Port : ActionPort  ActionPortLabel=if(u1 ==0)
  Constant : Constant  Value=360
  Constant1 : Constant  Value=100
  Constant2 : Constant  Value=128
  Constant3 : Constant  Value=360
  Constant4 : Constant
  Constant5 : Constant  Value=6.4
  Constant6 : Constant  Value=100
  Constant7 : Constant  Value=128
  Constant8 : Constant
  Constant9 : Constant  Value=6.4
  Divide{,1..3} (4 alike) : Product  Inputs=*/
  Minus : Sum  Inputs=+-
  Minus1 : Sum  Inputs=+-
  Product : Product
  Product1 : Product
  Sum : Sum  Inputs=|++
  Sum1 : Sum  Inputs=|++
  Out1 : Outport
  Out2 : Outport  Port=2
  wires:
  Product/1 -> Out1/1
  Constant/1 -> Product/1
  In1/1 -> Minus/1, Minus1/2
  Constant2/1 -> Minus/2
  Minus/1 -> Divide/1
  Constant5/1 -> Divide/2
  Divide/1 -> Divide1/1
  Constant1/1 -> Divide1/2
  Constant4/1 -> Sum/1
  Divide1/1 -> Sum/2
  Sum/1 -> Product/2
  Constant7/1 -> Minus1/1
  Minus1/1 -> Divide2/1
  Constant3/1 -> Product1/1
  Constant9/1 -> Divide2/2
  Divide2/1 -> Divide3/1
  Divide3/1 -> Sum1/2
  Product1/1 -> Out2/1
  Constant6/1 -> Divide3/2
  Sum1/1 -> Product1/2
  Constant8/1 -> Sum1/1

== system integratoin_2/Subsystem14/If Action Subsystem3 ==
  In1 : Inport
  In2 : Inport  Port=2
  In3 : Inport  Port=3
  In4 : Inport  Port=4
  Action Port : ActionPort  ActionPortLabel=else
  If : If  NumInputs=4  IfExpression=u1>10
  If Action Subsystem : Subsystem  TreatAsAtomicUnit=on
  If Action Subsystem1 : Subsystem  TreatAsAtomicUnit=on
  Merge : Merge
  Merge1 : Merge
  Out1 : Outport
  Out2 : Outport  Port=2
  wires:
  If/2 -> If Action Subsystem/Action
  In1/1 -> If/1
  In2/1 -> If/2
  In3/1 -> If/3
  In4/1 -> If/4
  If/1 -> If Action Subsystem1/Action
  If Action Subsystem1/1(Out1) -> Merge/1
  If Action Subsystem/1(Out1) -> Merge/2
  Merge/1 -> Out1/1
  If Action Subsystem1/2(Out2) -> Merge1/1
  If Action Subsystem/2(Out2) -> Merge1/2
  Merge1/1 -> Out2/1

== system integratoin_2/Subsystem15/Subsystem1 ==
  Data Type Conversion1 : DataTypeConversion  OutDataTypeStr=int32  SaturateOnIntegerOverflow=off  RndMeth=Floor
  Discrete Transfer Fcn : DiscreteTransferFcn  Numerator=num_Gd  Denominator=den_Gd
  Discrete Derivative : simulink/Discrete/Discrete Derivative  gainval=1.0  ICPrevScaledInput=0.0  OutMin=[]  OutMax=[]  OutDataType=fixdt(1, 16)  OutScaling=2^-10  DoSatur=off
  Display : Display
  Encoder : arduinosensorlib/Encoder  InputA=18  InputB=19  Mode=No reset  SampleTime=-1
  Gain1 : Gain  Gain=encoder_scale
  Gain2 : Gain  Gain=60/(2*pi)
  Out1 : Outport
  Out2 : Outport  Port=2
  wires:
  Gain1/1 -> Display/1, Gain2/1, Data Type Conversion1/1
  Encoder/1 -> Discrete Derivative/1
  Gain2/1 -> Out2/1
  Data Type Conversion1/1 -> Discrete Transfer Fcn/1
  Discrete Derivative/1 -> Gain1/1
  Discrete Transfer Fcn/1 -> Out1/1

== system integratoin_2/Subsystem15/Subsystem2 ==
  In2 : Inport
  Add : Sum  Commented=on  Inputs=+-
  Add1 : Sum  Commented=on
  Data Type Conversion : DataTypeConversion  OutDataTypeStr=uint8  SaturateOnIntegerOverflow=off  RndMeth=Floor
  Data Type Conversion1 : DataTypeConversion  OutDataTypeStr=double  SaturateOnIntegerOverflow=off  RndMeth=Floor
  Display1 : Display
  Gain : Gain  Commented=on  Gain=Kb
  Gain1 : Gain  Gain=255/Vlim
  PWM : arduinolib/PWM  pinNumber=11  frequencyType=Default  desiredFrequency=490.2  achievableFrequency=490.2
  Transfer Fcn : TransferFcn  Commented=on  Numerator=Km  Denominator=[L R]
  Transfer Fcn1 : TransferFcn  Commented=on  Numerator=1  Denominator=[J Kf]
  Out1 : Outport
  wires:
  ? -> Add/1
  ? -> Add1/1
  Add/1 -> Transfer Fcn/1
  Add1/1 -> Transfer Fcn1/1
  Transfer Fcn/1 -> Add1/2
  Gain/1 -> Add/2
  Transfer Fcn1/1 -> Gain/1
  In2/1 -> Gain1/1
  Gain1/1 -> Data Type Conversion/1
  Data Type Conversion1/1 -> Out1/1
  Data Type Conversion/1 -> Data Type Conversion1/1, Display1/1, PWM/1

== system integratoin_2/Subsystem15/Subsystem6 ==
  In1 : Inport
  Derivative2 : Derivative
  Gain1 : Gain  Gain=KI
  Gain2 : Gain  Gain=KP
  Gain3 : Gain  Gain=KD
  Integrator2 : Integrator
  Subtract2 : Sum  Inputs=+++
  Out1 : Outport
  wires:
  Gain1/1 -> Integrator2/1
  Gain2/1 -> Subtract2/2
  Integrator2/1 -> Subtract2/1
  In1/1 -> Gain2/1, Gain3/1, Gain1/1
  Derivative2/1 -> Subtract2/3
  Gain3/1 -> Derivative2/1
  Subtract2/1 -> Out1/1

== system integratoin_2/Subsystem16/Subsystem1 ==
  Data Type Conversion1 : DataTypeConversion  OutDataTypeStr=int32  SaturateOnIntegerOverflow=off  RndMeth=Floor
  Discrete Transfer Fcn : DiscreteTransferFcn  Numerator=num_Gd  Denominator=den_Gd
  Discrete Derivative : simulink/Discrete/Discrete Derivative  gainval=1.0  ICPrevScaledInput=0.0  OutMin=[]  OutMax=[]  OutDataType=fixdt(1, 16)  OutScaling=2^-10  DoSatur=off
  Display : Display
  Encoder : arduinosensorlib/Encoder  InputA=20  InputB=21  Mode=No reset  SampleTime=-1
  Gain1 : Gain  Gain=encoder_scale
  Gain2 : Gain  Gain=60/(2*pi)
  Out1 : Outport
  Out2 : Outport  Port=2
  wires:
  Gain1/1 -> Display/1, Gain2/1, Data Type Conversion1/1
  Encoder/1 -> Discrete Derivative/1
  Gain2/1 -> Out2/1
  Data Type Conversion1/1 -> Discrete Transfer Fcn/1
  Discrete Derivative/1 -> Gain1/1
  Discrete Transfer Fcn/1 -> Out1/1

== system integratoin_2/Subsystem16/Subsystem2 ==
  In2 : Inport
  Add : Sum  Commented=on  Inputs=+-
  Add1 : Sum  Commented=on
  Data Type Conversion : DataTypeConversion  OutDataTypeStr=uint8  SaturateOnIntegerOverflow=off  RndMeth=Floor
  Data Type Conversion1 : DataTypeConversion  OutDataTypeStr=double  SaturateOnIntegerOverflow=off  RndMeth=Floor
  Display1 : Display
  Gain : Gain  Commented=on  Gain=Kb
  Gain1 : Gain  Gain=255/Vlim
  PWM : arduinolib/PWM  pinNumber=3  frequencyType=Default  desiredFrequency=490.2  achievableFrequency=490.2
  Transfer Fcn : TransferFcn  Commented=on  Numerator=Km  Denominator=[L R]
  Transfer Fcn1 : TransferFcn  Commented=on  Numerator=1  Denominator=[J Kf]
  Out1 : Outport
  wires:
  ? -> Add/1
  ? -> Add1/1
  Add/1 -> Transfer Fcn/1
  Add1/1 -> Transfer Fcn1/1
  Transfer Fcn/1 -> Add1/2
  Gain/1 -> Add/2
  Transfer Fcn1/1 -> Gain/1
  In2/1 -> Gain1/1
  Gain1/1 -> Data Type Conversion/1
  Data Type Conversion1/1 -> Out1/1
  Data Type Conversion/1 -> Data Type Conversion1/1, Display1/1, PWM/1

== system integratoin_2/Subsystem16/Subsystem6 ==
  In1 : Inport
  Derivative2 : Derivative
  Gain1 : Gain  Gain=KI
  Gain2 : Gain  Gain=KP
  Gain3 : Gain  Gain=KD
  Integrator2 : Integrator
  Subtract2 : Sum  Inputs=+++
  Out1 : Outport
  wires:
  Gain1/1 -> Integrator2/1
  Gain2/1 -> Subtract2/2
  Integrator2/1 -> Subtract2/1
  In1/1 -> Gain2/1, Gain3/1, Gain1/1
  Derivative2/1 -> Subtract2/3
  Gain3/1 -> Derivative2/1
  Subtract2/1 -> Out1/1

== system integratoin_2/Subsystem2/Subsystem1 ==
  Data Type Conversion1 : DataTypeConversion  OutDataTypeStr=int32  SaturateOnIntegerOverflow=off  RndMeth=Floor
  Discrete Transfer Fcn : DiscreteTransferFcn  Numerator=num_Gd  Denominator=den_Gd
  Discrete Derivative : simulink/Discrete/Discrete Derivative  gainval=1.0  ICPrevScaledInput=0.0  OutMin=[]  OutMax=[]  OutDataType=fixdt(1, 16)  OutScaling=2^-10  DoSatur=off
  Display : Display
  Encoder : arduinosensorlib/Encoder  InputA=18  InputB=19  Mode=No reset  SampleTime=-1
  Gain1 : Gain  Gain=encoder_scale
  Gain2 : Gain  Gain=60/(2*pi)
  Out1 : Outport
  Out2 : Outport  Port=2
  wires:
  Gain1/1 -> Display/1, Gain2/1, Data Type Conversion1/1
  Encoder/1 -> Discrete Derivative/1
  Gain2/1 -> Out2/1
  Data Type Conversion1/1 -> Discrete Transfer Fcn/1
  Discrete Derivative/1 -> Gain1/1
  Discrete Transfer Fcn/1 -> Out1/1

== system integratoin_2/Subsystem2/Subsystem2 ==
  Data Type Conversion1 : DataTypeConversion  OutDataTypeStr=int32  SaturateOnIntegerOverflow=off  RndMeth=Floor
  Discrete Transfer Fcn : DiscreteTransferFcn  Numerator=num_Gd  Denominator=den_Gd
  Discrete Derivative : simulink/Discrete/Discrete Derivative  gainval=1.0  ICPrevScaledInput=0.0  OutMin=[]  OutMax=[]  OutDataType=fixdt(1, 16)  OutScaling=2^-10  DoSatur=off
  Display : Display
  Encoder : arduinosensorlib/Encoder  InputA=18  InputB=19  Mode=No reset  SampleTime=-1
  Gain1 : Gain  Gain=encoder_scale
  Gain2 : Gain  Gain=60/(2*pi)
  Out1 : Outport
  Out2 : Outport  Port=2
  wires:
  Gain1/1 -> Display/1, Gain2/1, Data Type Conversion1/1
  Encoder/1 -> Discrete Derivative/1
  Gain2/1 -> Out2/1
  Data Type Conversion1/1 -> Discrete Transfer Fcn/1
  Discrete Derivative/1 -> Gain1/1
  Discrete Transfer Fcn/1 -> Out1/1

== system integratoin_2/Subsystem2/Subsystem4 ==
  In1 : Inport
  Add : Sum  Inputs=+-
  Add1 : Sum
  Gain : Gain  Gain=Kb
  Transfer Fcn : TransferFcn  Numerator=Km  Denominator=[L R]
  Transfer Fcn1 : TransferFcn  Numerator=1  Denominator=[J Kf]
  Out1 : Outport
  wires:
  In1/1 -> Add/1
  ? -> Add1/1
  Add/1 -> Transfer Fcn/1
  Add1/1 -> Transfer Fcn1/1
  Transfer Fcn/1 -> Add1/2
  Gain/1 -> Add/2
  Transfer Fcn1/1 -> Gain/1, Out1/1

== system integratoin_2/Subsystem2/Subsystem5 ==
  In1 : Inport
  Derivative1 : Derivative
  Gain4 : Gain  Gain=KI
  Gain5 : Gain  Gain=KP
  Gain6 : Gain  Gain=KD
  Integrator1 : Integrator
  Subtract1 : Sum  Inputs=+++
  Out1 : Outport
  wires:
  Subtract1/1 -> Out1/1
  In1/1 -> Gain5/1, Gain6/1, Gain4/1
  Integrator1/1 -> Subtract1/1
  Derivative1/1 -> Subtract1/3
  Gain6/1 -> Derivative1/1
  Gain5/1 -> Subtract1/2
  Gain4/1 -> Integrator1/1

== system integratoin_2/light_Ctrl/Function-Call Subsystem1 ==
  function : TriggerPort  TriggerType=function-call  VariantControl=(inherit)
  Constant : Constant
  Constant1 : Constant  Value=3
  Delay : Delay  DelayLength=1
  Mod : Math  Operator=mod
  Sum : Sum  Inputs=|++
  Output : Outport
  wires:
  Constant/1 -> Sum/1
  Delay/1 -> Sum/2
  Constant1/1 -> Mod/2
  Sum/1 -> Delay/1, Mod/1
  Mod/1 -> Output/1

== system integratoin_2/light_Ctrl/If Action Subsystem ==
  Action Port : ActionPort  ActionPortLabel=if(u1 == 0)
  Constant : Constant
  Constant1 : Constant  Value=3
  Delay : Delay  DelayLength=1
  Mod : Math  Operator=mod
  Plus : Sum
  Out1 : Outport
  wires:
  Mod/1 -> Out1/1, Delay/1
  Constant/1 -> Plus/1
  Delay/1 -> Plus/2
  Plus/1 -> Mod/1
  Constant1/1 -> Mod/2

== system integratoin_2/light_Ctrl/Subsystem ==
  light1 : Inport
  sw3 : Inport  Port=2
  Drive_mode1 : Inport  Port=3
  Chart1 : Stateflow chart  TreatAsAtomicUnit=on
  Subsystem : Subsystem
  light_mode : Outport
  wires:
  Chart1/1(light_mode) -> Subsystem/2(light_mode), light_mode/1
  light1/1 -> Subsystem/1(light)
  sw3/1 -> Chart1/1(sw3)
  Drive_mode1/1 -> Chart1/2(Drive_mode)

== system integratoin_2/State_Ctrl/ADAS_state/If Action Subsystem ==
  sw2 : Inport
  Action Port : ActionPort  ActionPortLabel=if(u1 ==1)
  Chart : Stateflow chart  TreatAsAtomicUnit=on
  ADAS_state : Outport
  wires:
  sw2/1 -> Chart/1(sw2)
  Chart/1(ADAS_state) -> ADAS_state/1

== system integratoin_2/State_Ctrl/ADAS_state/If Action Subsystem1 ==
  Action Port : ActionPort  ActionPortLabel=if(u1 == 0)
  Constant2 : Constant
  Constant3 : Constant  Value=2
  Delay1 : Delay  DelayLength=1  InitialCondition=0
  Mod1 : Math  Operator=mod
  Sum : Sum  Inputs=|++
  sw2 : Outport
  wires:
  Mod1/1 -> sw2/1
  Delay1/1 -> Sum/2
  Constant3/1 -> Mod1/2
  Sum/1 -> Delay1/1, Mod1/1
  Constant2/1 -> Sum/1

== system integratoin_2/State_Ctrl/ADAS_state/SW2 ==
  function : TriggerPort  TriggerType=function-call  VariantControl=(inherit)
  Constant : Constant
  Constant1 : Constant  Value=2
  Delay : Delay  DelayLength=1  InitialCondition=0
  Mod : Math  Operator=mod
  Sum : Sum  Inputs=|++
  SW2 : Outport
  wires:
  Sum/1 -> Delay/1, Mod/1
  Constant1/1 -> Mod/2
  Mod/1 -> SW2/1
  Constant/1 -> Sum/1
  Delay/1 -> Sum/2

== system integratoin_2/State_Ctrl/drive_mode/SW1 ==
  function : TriggerPort  TriggerType=function-call  VariantControl=(inherit)
  Constant : Constant
  Constant1 : Constant  Value=2
  Delay : Delay  DelayLength=1
  Mod : Math  Operator=mod
  Sum : Sum  Inputs=|++
  Output : Outport
  wires:
  Constant/1 -> Sum/1
  Sum/1 -> Delay/1, Mod/1
  Constant1/1 -> Mod/2
  Delay/1 -> Sum/2
  Mod/1 -> Output/1

== system integratoin_2/Subsystem14/If Action Subsystem3/If Action Subsystem ==
  Action Port : ActionPort  ActionPortLabel=else
  Constant : Constant  Value=0
  Constant1 : Constant  Value=0
  Out1 : Outport
  Out2 : Outport  Port=2
  wires:
  Constant1/1 -> Out2/1
  Constant/1 -> Out1/1

== system integratoin_2/Subsystem14/If Action Subsystem3/If Action Subsystem1 ==
  Action Port : ActionPort  ActionPortLabel=if(u1>10)
  Constant : Constant  Value=360
  Constant1 : Constant  Value=360
  Out1 : Outport
  Out2 : Outport  Port=2
  wires:
  Constant/1 -> Out1/1
  Constant1/1 -> Out2/1

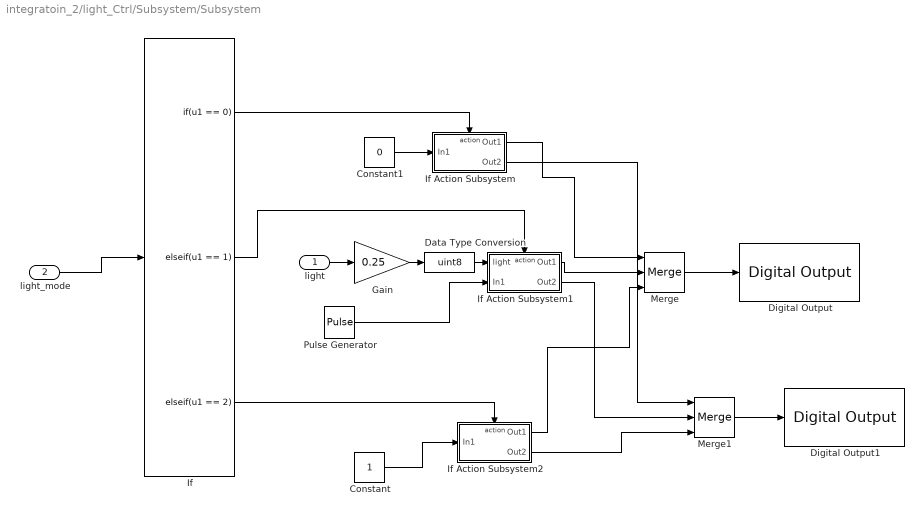
== system integratoin_2/light_Ctrl/Subsystem/Subsystem ==
  light : Inport
  light_mode : Inport  Port=2
  Constant : Constant
  Constant1 : Constant  Value=0
  Data Type Conversion : DataTypeConversion  OutDataTypeStr=uint8  SaturateOnIntegerOverflow=off  RndMeth=Floor
  Digital Output : arduinolib/Digital Output  pinNumber=LED2_R  Direction=output  blockPlatform=arduino
  Digital Output1 : arduinolib/Digital Output  pinNumber=LED2_B  Direction=output  blockPlatform=arduino
  Gain : Gain  Gain=0.25
  If : If  IfExpression=u1 == 0  ElseIfExpressions=u1 == 1, u1 == 2  ShowElse=off
  If Action Subsystem : Subsystem  TreatAsAtomicUnit=on
  If Action Subsystem1 : Subsystem  TreatAsAtomicUnit=on
  If Action Subsystem2 : Subsystem  TreatAsAtomicUnit=on
  Merge : Merge  Inputs=3
  Merge1 : Merge  Inputs=3
  Pulse Generator : DiscretePulseGenerator  PulseType=Time based  Period=0.2  PulseWidth=50
  wires:
  light_mode/1 -> If/1
  If/1 -> If Action Subsystem/Action
  If/2 -> If Action Subsystem1/Action
  If/3 -> If Action Subsystem2/Action
  Constant1/1 -> If Action Subsystem/1(In1)
  Constant/1 -> If Action Subsystem2/1(In1)
  If Action Subsystem/1(Out1) -> Merge/1
  If Action Subsystem1/1(Out1) -> Merge/2
  If Action Subsystem2/1(Out1) -> Merge/3
  Merge/1 -> Digital Output/1
  light/1 -> Gain/1
  Gain/1 -> Data Type Conversion/1
  Data Type Conversion/1 -> If Action Subsystem1/1(light)
  Pulse Generator/1 -> If Action Subsystem1/2(In1)
  If Action Subsystem1/2(Out2) -> Merge1/2
  If Action Subsystem/2(Out2) -> Merge1/1
  If Action Subsystem2/2(Out2) -> Merge1/3
  Merge1/1 -> Digital Output1/1

== system integratoin_2/light_Ctrl/Subsystem/Subsystem/If Action Subsystem ==
  In1 : Inport
  Action Port : ActionPort  ActionPortLabel=if(u1 == 0)
  Out1 : Outport
  Out2 : Outport  Port=2
  wires:
  In1/1 -> Out2/1, Out1/1

== system integratoin_2/light_Ctrl/Subsystem/Subsystem/If Action Subsystem1 ==
  light : Inport
  In1 : Inport  Port=2
  Action Port : ActionPort  ActionPortLabel=elseif(u1 == 1)
  Constant : Constant
  Constant1 : Constant  Value=0
  If : If  IfExpression=u1 <= 150
  If Action Subsystem : Subsystem  TreatAsAtomicUnit=on
  If Action Subsystem1 : Subsystem  TreatAsAtomicUnit=on
  Merge : Merge
  Out1 : Outport
  Out2 : Outport  Port=2
  wires:
  light/1 -> If/1
  Constant/1 -> If Action Subsystem/1(In1)
  Constant1/1 -> If Action Subsystem1/1(In1)
  If/1 -> If Action Subsystem/Action
  If/2 -> If Action Subsystem1/Action
  If Action Subsystem/1(Out1) -> Merge/1
  If Action Subsystem1/1(Out1) -> Merge/2
  Merge/1 -> Out1/1
  In1/1 -> Out2/1

== system integratoin_2/light_Ctrl/Subsystem/Subsystem/If Action Subsystem2 ==
  In1 : Inport
  Action Port : ActionPort  ActionPortLabel=elseif( u1 == 2)
  Out1 : Outport
  Out2 : Outport  Port=2
  wires:
  In1/1 -> Out2/1, Out1/1

== system integratoin_2/light_Ctrl/Subsystem/Subsystem/If Action Subsystem1/If Action Subsystem ==
  In1 : Inport
  Action Port : ActionPort  ActionPortLabel=if(u1 <= 150)
  Out1 : Outport
  wires:
  In1/1 -> Out1/1

== system integratoin_2/light_Ctrl/Subsystem/Subsystem/If Action Subsystem1/If Action Subsystem1 ==
  In1 : Inport
  Action Port : ActionPort  ActionPortLabel=else
  Out1 : Outport
  wires:
  In1/1 -> Out1/1
